simulink subsystem "CoolingControlRing_subsysref"  (R2020a)
settings: Solver=VariableStepAuto  StartTime=0.0  StopTime=10.0  RelTol=1e-3
libraries: inverter_loop_pump_and_fan_PWM_LVLibrary x1, motor_loop_pump_and_fan_PWM_LVLibrary x1, pump_and_fans_workingLibrary x1, inverter_loop_pump_and_fan_PWMLibrary x1, motor_loop_pump_and_fan_PWMLibrary x1, All_Sensors_Working x1
settings Model: Creator=Kiera  LastModifiedBy=Kiera

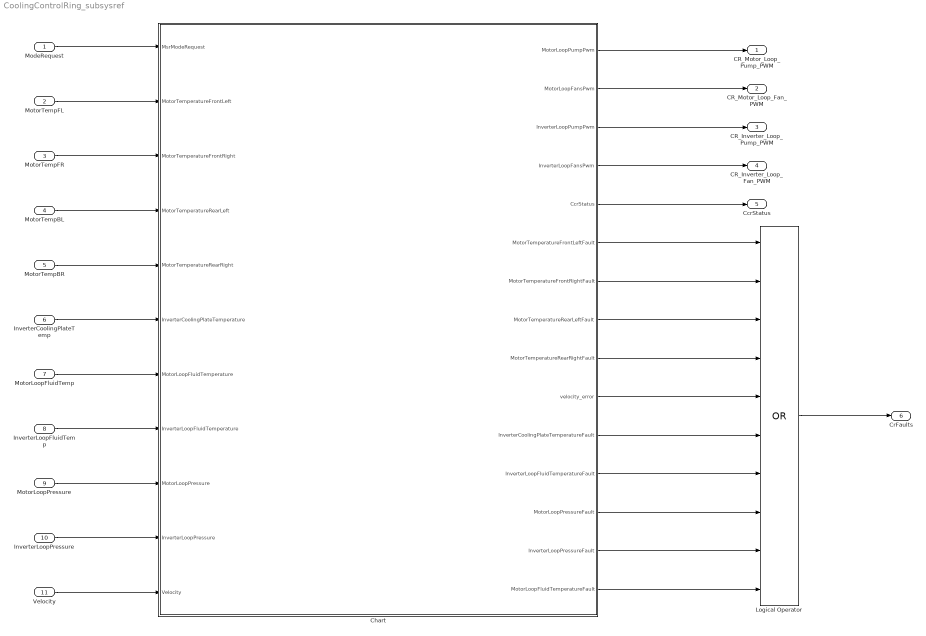
== system CoolingControlRing_subsysref ==
  ModeRequest : Inport
  MotorTempFL : Inport  Port=2
  MotorTempFR : Inport  Port=3
  MotorTempBL : Inport  Port=4
  MotorTempBR : Inport  Port=5
  InverterCoolingPlateTemp : Inport  Port=6
  MotorLoopFluidTemp : Inport  Port=7
  InverterLoopFluidTemp : Inport  Port=8
  MotorLoopPressure : Inport  Port=9
  InverterLoopPressure : Inport  Port=10
  Velocity : Inport  Port=11
  Chart : Stateflow chart  RequirementInfo={} %GIDa_8f277666_618f_4999_b577_53313bd8b4b0  TreatAsAtomicUnit=on
  Logical Operator : Logic  Operator=OR  Inputs=10  AllPortsSameDT=off  OutDataTypeStr=boolean
  CR_Motor_Loop_Pump_PWM : Outport  VectorParamsAs1DForOutWhenUnconnected=off
  CR_Motor_Loop_Fan_PWM : Outport  Port=2  VectorParamsAs1DForOutWhenUnconnected=off
  CR_Inverter_Loop_Pump_PWM : Outport  Port=3  VectorParamsAs1DForOutWhenUnconnected=off
  CR_Inverter_Loop_Fan_PWM : Outport  Port=4  VectorParamsAs1DForOutWhenUnconnected=off
  CcrStatus : Outport  Port=5  VectorParamsAs1DForOutWhenUnconnected=off
  CrFaults : Outport  Port=6  VectorParamsAs1DForOutWhenUnconnected=off
  wires:
  Chart/15(MotorLoopFluidTemperatureFault) -> Logical Operator/10
  Logical Operator/1 -> CrFaults/1
  MotorLoopFluidTemp/1 -> Chart/7(MotorLoopFluidTemperature)
  Chart/10(velocity_error) -> Logical Operator/5
  Chart/11(InverterCoolingPlateTemperatureFault) -> Logical Operator/6
  Chart/13(MotorLoopPressureFault) -> Logical Operator/8
  InverterCoolingPlateTemp/1 -> Chart/6(InverterCoolingPlateTemperature)
  Chart/12(InverterLoopFluidTemperatureFault) -> Logical Operator/7
  Chart/6(MotorTemperatureFrontLeftFault) -> Logical Operator/1
  ModeRequest/1 -> Chart/1(MsrModeRequest)
  MotorTempBL/1 -> Chart/4(MotorTemperatureRearLeft)
  Chart/3(InverterLoopPumpPwm) -> CR_Inverter_Loop_Pump_PWM/1
  Chart/2(MotorLoopFansPwm) -> CR_Motor_Loop_Fan_PWM/1
  InverterLoopPressure/1 -> Chart/10(InverterLoopPressure)
  MotorTempBR/1 -> Chart/5(MotorTemperatureRearRight)
  Chart/8(MotorTemperatureRearLeftFault) -> Logical Operator/3
  MotorTempFL/1 -> Chart/2(MotorTemperatureFrontLeft)
  Chart/1(MotorLoopPumpPwm) -> CR_Motor_Loop_Pump_PWM/1
  Chart/14(InverterLoopPressureFault) -> Logical Operator/9
  Chart/4(InverterLoopFansPwm) -> CR_Inverter_Loop_Fan_PWM/1
  Chart/5(CcrStatus) -> CcrStatus/1
  Chart/9(MotorTemperatureRearRightFault) -> Logical Operator/4
  InverterLoopFluidTemp/1 -> Chart/8(InverterLoopFluidTemperature)
  MotorTempFR/1 -> Chart/3(MotorTemperatureFrontRight)
  Chart/7(MotorTemperatureFrontRightFault) -> Logical Operator/2
  MotorLoopPressure/1 -> Chart/9(MotorLoopPressure)
  Velocity/1 -> Chart/11(Velocity)

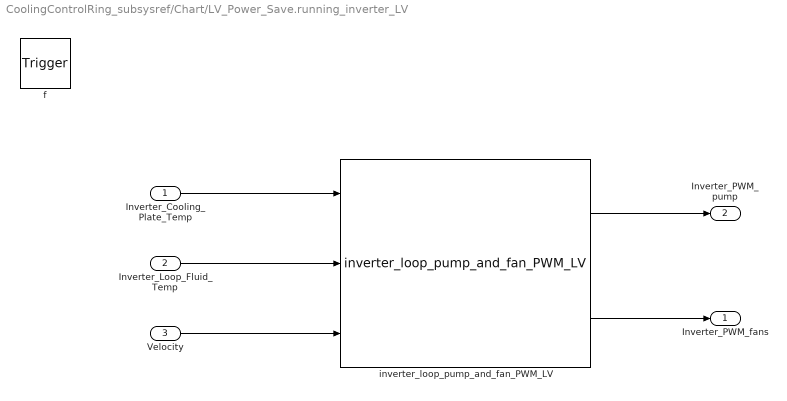
== system CoolingControlRing_subsysref/Chart/LV_Power_Save.running_inverter_LV ==
  Inverter_Cooling_Plate_Temp : Inport  OutDataTypeStr=double  PortDimensions=1
  Inverter_Loop_Fluid_Temp : Inport  Port=2  OutDataTypeStr=double  PortDimensions=1
  Velocity : Inport  Port=3  OutDataTypeStr=double  PortDimensions=1
  f : TriggerPort  TriggerType=function-call  VariantControl=Variant
      settings: CopyFcn=Stateflow.SLINSF.SimulinkMan.removeBlockPreDeleteFcn  PreDeleteFcn=Stateflow.SLINSF.SimulinkMan.unsafePredeleteFcn
  inverter_loop_pump_and_fan_PWM_LV : inverter_loop_pump_and_fan_PWM_LVLibrary/inverter_loop_pump_and_fan_PWM_LV  SystemSampleTime=-1  Latency=0  AutoFrameSizeCalculation=off
  Inverter_PWM_fans : Outport  VectorParamsAs1DForOutWhenUnconnected=off
  Inverter_PWM_pump : Outport  Port=2  VectorParamsAs1DForOutWhenUnconnected=off
  wires:
  inverter_loop_pump_and_fan_PWM_LV/2 -> Inverter_PWM_fans/1
  inverter_loop_pump_and_fan_PWM_LV/1 -> Inverter_PWM_pump/1
  Velocity/1 -> inverter_loop_pump_and_fan_PWM_LV/3
  Inverter_Cooling_Plate_Temp/1 -> inverter_loop_pump_and_fan_PWM_LV/1
  Inverter_Loop_Fluid_Temp/1 -> inverter_loop_pump_and_fan_PWM_LV/2

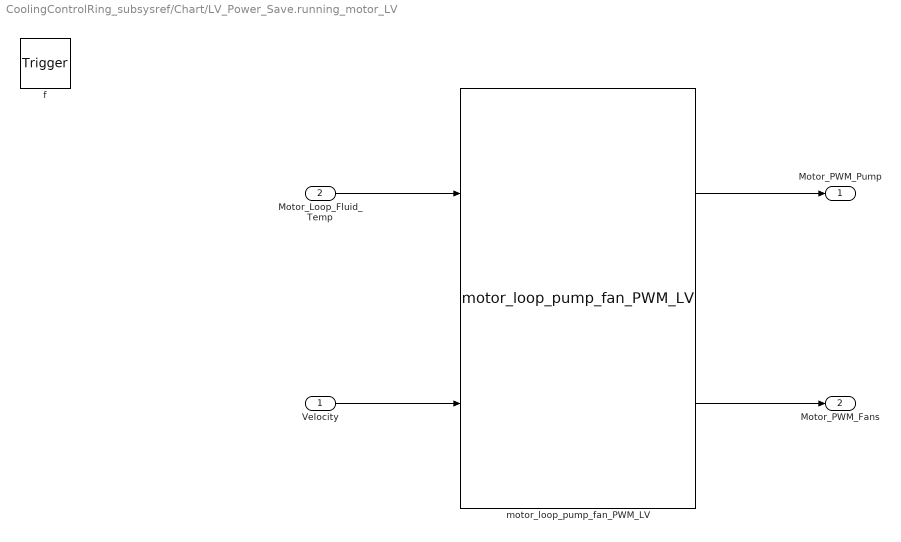
== system CoolingControlRing_subsysref/Chart/LV_Power_Save.running_motor_LV ==
  Velocity : Inport  OutDataTypeStr=double  PortDimensions=1
  Motor_Loop_Fluid_Temp : Inport  Port=2  OutDataTypeStr=double  PortDimensions=1
  f : TriggerPort  TriggerType=function-call  VariantControl=Variant
      settings: CopyFcn=Stateflow.SLINSF.SimulinkMan.removeBlockPreDeleteFcn  PreDeleteFcn=Stateflow.SLINSF.SimulinkMan.unsafePredeleteFcn
  motor_loop_pump_fan_PWM_LV : motor_loop_pump_and_fan_PWM_LVLibrary/motor_loop_pump_fan_PWM_LV  SystemSampleTime=-1  Latency=0  AutoFrameSizeCalculation=off
  Motor_PWM_Pump : Outport  OutDataTypeStr=double  PortDimensions=1  VectorParamsAs1DForOutWhenUnconnected=off
  Motor_PWM_Fans : Outport  Port=2  OutDataTypeStr=double  PortDimensions=1  VectorParamsAs1DForOutWhenUnconnected=off
  wires:
  Velocity/1 -> motor_loop_pump_fan_PWM_LV/2
  Motor_Loop_Fluid_Temp/1 -> motor_loop_pump_fan_PWM_LV/1
  motor_loop_pump_fan_PWM_LV/2 -> Motor_PWM_Fans/1
  motor_loop_pump_fan_PWM_LV/1 -> Motor_PWM_Pump/1

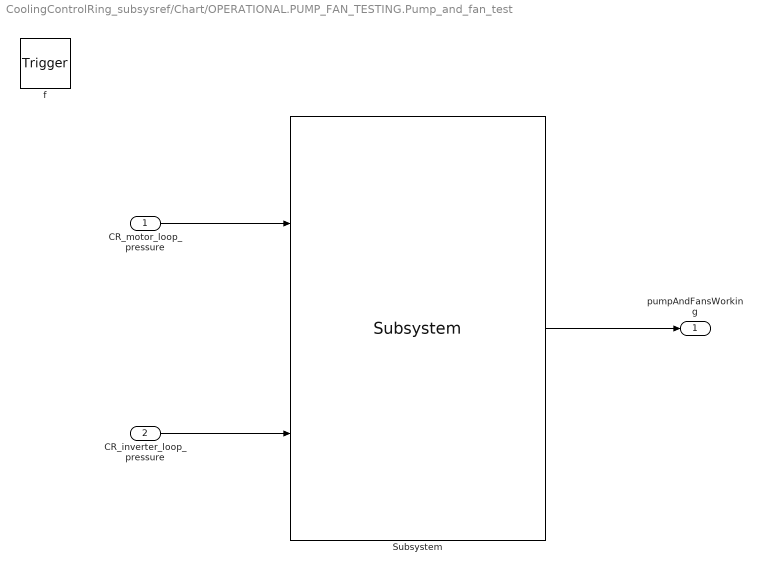
== system CoolingControlRing_subsysref/Chart/OPERATIONAL.PUMP_FAN_TESTING.Pump_and_fan_test ==
  CR_motor_loop_pressure : Inport  OutDataTypeStr=double  PortDimensions=1
  CR_inverter_loop_pressure : Inport  Port=2  OutDataTypeStr=double  PortDimensions=1
  f : TriggerPort  TriggerType=function-call  VariantControl=Variant
      settings: CopyFcn=Stateflow.SLINSF.SimulinkMan.removeBlockPreDeleteFcn  PreDeleteFcn=Stateflow.SLINSF.SimulinkMan.unsafePredeleteFcn
  Subsystem : pump_and_fans_workingLibrary/Subsystem  SystemSampleTime=-1  Latency=0  AutoFrameSizeCalculation=off
  pumpAndFansWorking : Outport  VectorParamsAs1DForOutWhenUnconnected=off
  wires:
  Subsystem/1 -> pumpAndFansWorking/1
  CR_inverter_loop_pressure/1 -> Subsystem/2
  CR_motor_loop_pressure/1 -> Subsystem/1

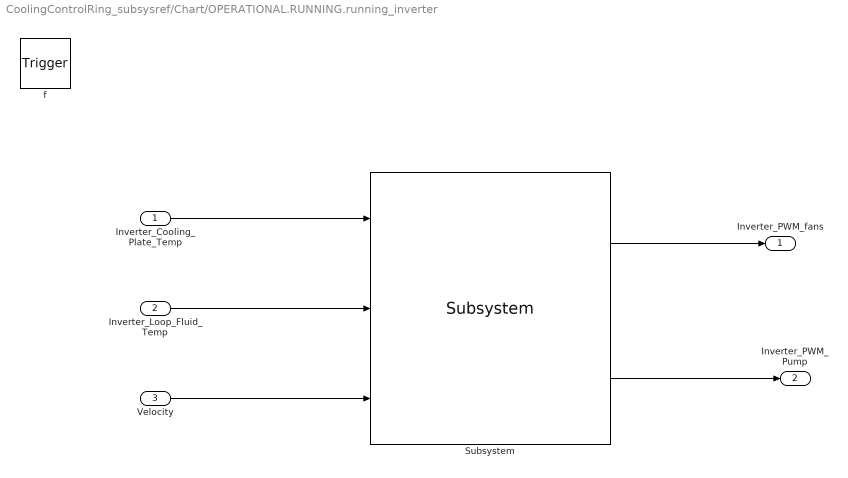
== system CoolingControlRing_subsysref/Chart/OPERATIONAL.RUNNING.running_inverter ==
  Inverter_Cooling_Plate_Temp : Inport  OutDataTypeStr=double  PortDimensions=1
  Inverter_Loop_Fluid_Temp : Inport  Port=2  OutDataTypeStr=double  PortDimensions=1
  Velocity : Inport  Port=3  OutDataTypeStr=double  PortDimensions=1
  f : TriggerPort  TriggerType=function-call  VariantControl=Variant
      settings: CopyFcn=Stateflow.SLINSF.SimulinkMan.removeBlockPreDeleteFcn  PreDeleteFcn=Stateflow.SLINSF.SimulinkMan.unsafePredeleteFcn
  Subsystem : inverter_loop_pump_and_fan_PWMLibrary/Subsystem  SystemSampleTime=-1  Latency=0  AutoFrameSizeCalculation=off
  Inverter_PWM_fans : Outport  OutDataTypeStr=double  PortDimensions=1  VectorParamsAs1DForOutWhenUnconnected=off
  Inverter_PWM_Pump : Outport  Port=2  OutDataTypeStr=double  PortDimensions=1  VectorParamsAs1DForOutWhenUnconnected=off
  wires:
  Subsystem/1 -> Inverter_PWM_fans/1
  Subsystem/2 -> Inverter_PWM_Pump/1
  Velocity/1 -> Subsystem/3
  Inverter_Loop_Fluid_Temp/1 -> Subsystem/2
  Inverter_Cooling_Plate_Temp/1 -> Subsystem/1

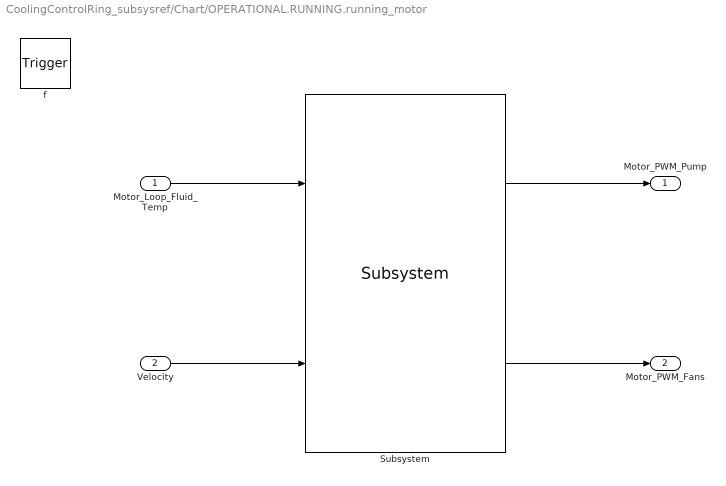
== system CoolingControlRing_subsysref/Chart/OPERATIONAL.RUNNING.running_motor ==
  Motor_Loop_Fluid_Temp : Inport  OutDataTypeStr=double  PortDimensions=1
  Velocity : Inport  Port=2  OutDataTypeStr=double  PortDimensions=1
  f : TriggerPort  TriggerType=function-call  VariantControl=Variant
      settings: CopyFcn=Stateflow.SLINSF.SimulinkMan.removeBlockPreDeleteFcn  PreDeleteFcn=Stateflow.SLINSF.SimulinkMan.unsafePredeleteFcn
  Subsystem : motor_loop_pump_and_fan_PWMLibrary/Subsystem  SystemSampleTime=-1  Latency=0  AutoFrameSizeCalculation=off
  Motor_PWM_Pump : Outport  OutDataTypeStr=double  PortDimensions=1  VectorParamsAs1DForOutWhenUnconnected=off
  Motor_PWM_Fans : Outport  Port=2  OutDataTypeStr=double  PortDimensions=1  VectorParamsAs1DForOutWhenUnconnected=off
  wires:
  Motor_Loop_Fluid_Temp/1 -> Subsystem/1
  Velocity/1 -> Subsystem/2
  Subsystem/2 -> Motor_PWM_Fans/1
  Subsystem/1 -> Motor_PWM_Pump/1

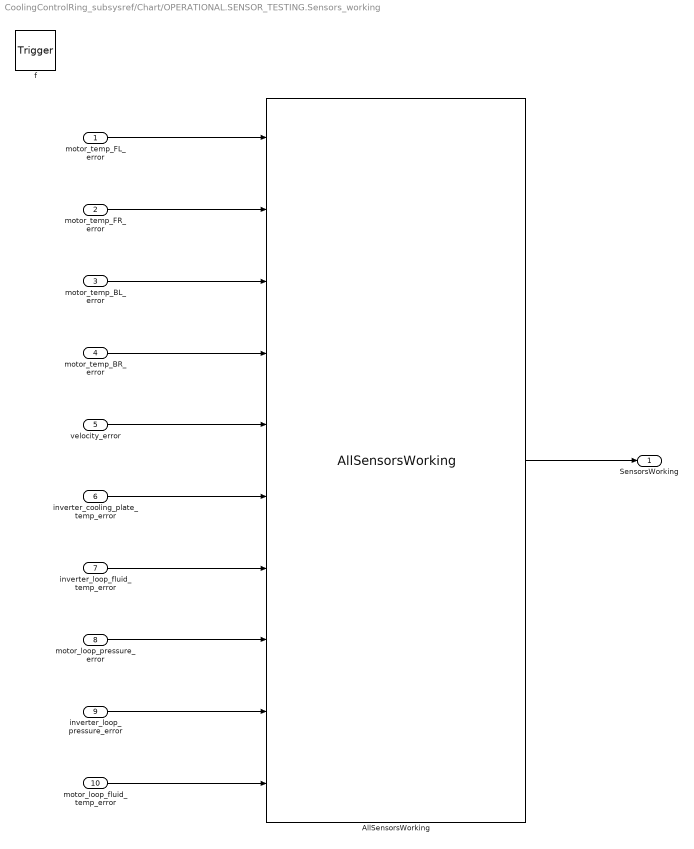
== system CoolingControlRing_subsysref/Chart/OPERATIONAL.SENSOR_TESTING.Sensors_working ==
  motor_temp_FL_error : Inport  OutDataTypeStr=double  PortDimensions=1
  motor_temp_FR_error : Inport  Port=2  OutDataTypeStr=double  PortDimensions=1
  motor_temp_BL_error : Inport  Port=3  OutDataTypeStr=double  PortDimensions=1
  motor_temp_BR_error : Inport  Port=4  OutDataTypeStr=double  PortDimensions=1
  velocity_error : Inport  Port=5  OutDataTypeStr=double  PortDimensions=1
  inverter_cooling_plate_temp_error : Inport  Port=6  OutDataTypeStr=double  PortDimensions=1
  inverter_loop_fluid_temp_error : Inport  Port=7  OutDataTypeStr=double  PortDimensions=1
  motor_loop_pressure_error : Inport  Port=8  OutDataTypeStr=double  PortDimensions=1
  inverter_loop_pressure_error : Inport  Port=9  OutDataTypeStr=double  PortDimensions=1
  motor_loop_fluid_temp_error : Inport  Port=10  OutDataTypeStr=double  PortDimensions=1
  f : TriggerPort  TriggerType=function-call  VariantControl=Variant
      settings: CopyFcn=Stateflow.SLINSF.SimulinkMan.removeBlockPreDeleteFcn  PreDeleteFcn=Stateflow.SLINSF.SimulinkMan.unsafePredeleteFcn
  AllSensorsWorking : All_Sensors_Working/AllSensorsWorking  SystemSampleTime=-1  Latency=0  AutoFrameSizeCalculation=off
  SensorsWorking : Outport  VectorParamsAs1DForOutWhenUnconnected=off
  wires:
  motor_loop_fluid_temp_error/1 -> AllSensorsWorking/10
  inverter_loop_pressure_error/1 -> AllSensorsWorking/9
  motor_loop_pressure_error/1 -> AllSensorsWorking/8
  inverter_loop_fluid_temp_error/1 -> AllSensorsWorking/7
  inverter_cooling_plate_temp_error/1 -> AllSensorsWorking/6
  velocity_error/1 -> AllSensorsWorking/5
  motor_temp_BR_error/1 -> AllSensorsWorking/4
  motor_temp_BL_error/1 -> AllSensorsWorking/3
  motor_temp_FL_error/1 -> AllSensorsWorking/1
  motor_temp_FR_error/1 -> AllSensorsWorking/2
  AllSensorsWorking/1 -> SensorsWorking/1

== stateflow chart CoolingControlRing_subsysref/Chart ==
  state OFF
    entry:
    MotorLoopPumpPwm=0;
    MotorLoopFansPwm=0;
    InverterLoopPumpPwm=0;
    InverterLoopFansPwm=0;
    CcrStatus = RING_STATUS.OFF;
    SensorSanity;
  state SHUTDOWN
    entry:
    CcrStatus = RING_STATUS.SHUTDOWN_COMPLETE_LV;
    % shutdown cooling fans and pump
  state OPERATIONAL
    entry:
    CcrStatus = RING_STATUS.SHUTDOWN_IN_PROGRESS_LV;
    state RUNNING
      entry:
      CcrStatus = RING_STATUS.RUNNING;
      during:
      [MotorLoopPumpPwm,MotorLoopFansPwm] = running_motor(MotorLoopFluidTemperature,Velocity)
      [InverterLoopFansPwm,InverterLoopPumpPwm] = running_inverter(InverterCoolingPlateTemperature,InverterLoopFluidTemperature,Velocity)
      state [Motor_PWM_Pump,Motor_PWM_Fans] = running_motor(Motor_Loop_Fluid_Temp,Velocity) [function]
      state [Inverter_PWM_fans,Inverter_PWM_Pump] = running_inverter(Inverter_Cooling_Plate_Temp,Inverter_Loop_Fluid_Temp,Velocity) [function]
    state TestingComplete
      entry:
      CcrStatus = RING_STATUS.STARTUP_COMPLETE_LV;
    state SENSOR_TESTING
      % sanity test on signal inputs
      % ensure sensor output values are within reasonable range
      entry:
      sensorsWorking=0;
      during:
      SensorSanity;
      sensorsWorking = Sensors_working(MotorTemperatureFrontLeftFault,MotorTemperatureFrontRightFault,MotorTemperatureRearLeftFault,MotorTemperatureRearRightFault,velocity_error,InverterCoolingPlateTemperatureFault,MotorLoopFluidTemperatureFault,InverterLoopFluidTemperatureFault,MotorLoopPressureFault,InverterLoopPressureFault);
      state SensorsWorking = Sensors_working(motor_temp_FL_error,motor_temp_FR_error,motor_temp_BL_error,motor_temp_BR_error,velocity_error,inverter_cooling_plate_temp_error,inverter_loop_fluid_temp_error,motor_loop_pressure_error,inverter_loop_pressure_error,motor_loop_fluid_temp_error) [function]
    state PUMP_FAN_TESTING
      % turning pump on and ensuring pressure ~=0
      % turning fans on and ensuring RPM ~=0
      entry:
      pumpAndFansWorking = 0;
      MotorLoopPumpPwm = CR.Motor_Testing_PWM_Pump;
      MotorLoopFansPwm = CR.Motor_Testing_PWM_Fans;
      InverterLoopPumpPwm = CR.Inverter_Testing_PWM_Pump;
      InverterLoopFansPwm = CR.Inverter_Testing_PWM_Fans;
      during:
      pumpAndFansWorking = Pump_and_fan_test(MotorLoopPressure,InverterLoopPressure)
      state pumpAndFansWorking = Pump_and_fan_test(CR_motor_loop_pressure,CR_inverter_loop_pressure) [function]
    (default) -> SENSOR_TESTING
    TestingComplete -> RUNNING : [MsrModeRequest == MSR_REQUEST.RUNNING]
    SENSOR_TESTING -> PUMP_FAN_TESTING : [sensorsWorking == 1]
    PUMP_FAN_TESTING -> TestingComplete : [pumpAndFansWorking == 1]
  state LV_Power_Save [commented out]
    entry:
    CcrStatus = CR.State.Running_LV;
    during:
    [MotorLoopPumpPwm,MotorLoopFansPwm] = running_motor_LV(Velocity,MotorLoopFluidTemperature)
    [InverterLoopFansPwm,InverterLoopPumpPwm] = running_inverter_LV(InverterCoolingPlateTemperature,InverterLoopFluidTemperature,Velocity)
    state [Motor_PWM_Pump,Motor_PWM_Fans] = running_motor_LV(Velocity,Motor_Loop_Fluid_Temp) [function] [commented out]
    state [Inverter_PWM_fans,Inverter_PWM_pump] = running_inverter_LV(Inverter_Cooling_Plate_Temp,Inverter_Loop_Fluid_Temp,Velocity) [function] [commented out]
  (default) -> OFF
  SHUTDOWN -> OFF : [MsrModeRequest == MSR_REQUEST.OFF]
  OPERATIONAL -> SHUTDOWN : [MsrModeRequest == MSR_REQUEST.SHUTDOWN_LV]
  OFF -> OPERATIONAL : [MsrModeRequest == MSR_REQUEST.STARTUP_LV]
  data: Motor_Loop_Fluid_Temp function_input double size=1; Velocity function_input double size=1; Motor_PWM_Pump function_output double size=1; Motor_PWM_Fans function_output double size=1; Inverter_Cooling_Plate_Temp function_input double size=1; Inverter_Loop_Fluid_Temp function_input double size=1; Velocity function_input double size=1; Inverter_PWM_fans function_output double size=1; Inverter_PWM_Pump function_output double size=1; SensorsWorking function_output; motor_temp_FL_error function_input double size=1; motor_temp_FR_error function_input double size=1; motor_temp_BL_error function_input double size=1; motor_temp_BR_error function_input double size=1; velocity_error function_input double size=1; inverter_cooling_plate_temp_error function_input double size=1; inverter_loop_fluid_temp_error function_input double size=1; motor_loop_pressure_error function_input double size=1; inverter_loop_pressure_error function_input double size=1; motor_loop_fluid_temp_error function_input double size=1; CR_motor_loop_pressure function_input double size=1; CR_inverter_loop_pressure function_input double size=1; pumpAndFansWorking function_output; Velocity function_input double size=1; Motor_PWM_Pump function_output double size=1; Motor_PWM_Fans function_output double size=1; Motor_Loop_Fluid_Temp function_input double size=1; Inverter_Cooling_Plate_Temp function_input double size=1; Inverter_Loop_Fluid_Temp function_input double size=1; Velocity function_input double size=1; Inverter_PWM_fans function_output double size=1; Inverter_PWM_pump function_output double size=1; MsrModeRequest input Enum: MSR_REQUEST; MotorLoopPumpPwm output double; MotorLoopFansPwm output double; InverterLoopPumpPwm output; InverterLoopFansPwm output; MotorTemperatureFrontLeft input; MotorTemperatureFrontRight input; MotorTemperatureRearLeft input; MotorTemperatureRearRight input; InverterCoolingPlateTemperature input; MotorLoopFluidTemperature input; InverterLoopFluidTemperature input; MotorLoopPressure input; InverterLoopPressure input; Velocity input; CcrStatus output Enum: RING_STATUS; CR parameter; MotorTemperatureFrontLeftFault output; MotorTemperatureFrontRightFault output; MotorTemperatureRearLeftFault output; MotorTemperatureRearRightFault output; velocity_error output; InverterCoolingPlateTemperatureFault output; InverterLoopFluidTemperatureFault output; MotorLoopPressureFault output; InverterLoopPressureFault output; sensorsWorking local; pumpAndFansWorking local; MotorLoopFluidTemperatureFault output
  function SensorSanity:
    | function SensorSanity
    | if (MotorTemperatureFrontLeft > CR.motor_temp_max || MotorTemperatureFrontLeft < CR.motor_temp_min)
    |     MotorTemperatureFrontLeftFault = CR.ERROR.FAILURE;
    | else
    |     MotorTemperatureFrontLeftFault = CR.ERROR.PASS;
    | end
    | 
    | if (MotorTemperatureFrontRight > CR.motor_temp_max || MotorTemperatureFrontRight < CR.motor_temp_min)
    |     MotorTemperatureFrontRightFault = CR.ERROR.FAILURE;
    | else
    |     MotorTemperatureFrontRightFault = CR.ERROR.PASS;
    | end
    | 
    | if (MotorTemperatureRearLeft > CR.motor_temp_max || MotorTemperatureRearLeft < CR.motor_temp_min)
    |     MotorTemperatureRearLeftFault = CR.ERROR.FAILURE;
    | else
    |     MotorTemperatureRearLeftFault = CR.ERROR.PASS;
    | end
    | 
    | if (MotorTemperatureRearRight > CR.motor_temp_max || MotorTemperatureRearRight < CR.motor_temp_min)
    |     MotorTemperatureRearRightFault = CR.ERROR.FAILURE;
    | else
    |     MotorTemperatureRearRightFault = CR.ERROR.PASS;
    | end
    | 
    | if (Velocity > CR.velocity_max || Velocity < CR.velocity_min)
    |     velocity_error = CR.ERROR.FAILURE;
    | else
    |     velocity_error = CR.ERROR.PASS;
    | end
    | 
    | if (InverterCoolingPlateTemperature > CR.inverter_cooling_plate_max || InverterCoolingPlateTemperature < CR.inverter_cooling_plate_min)
    |     InverterCoolingPlateTemperatureFault = CR.ERROR.FAILURE;
    | else
    |     InverterCoolingPlateTemperatureFault = CR.ERROR.PASS;
    | end
    | 
    | if (MotorLoopFluidTemperature > CR.motor_fluid_temp_max || MotorLoopFluidTemperature < CR.motor_fluid_temp_min)
    |     MotorLoopFluidTemperatureFault = CR.ERROR.FAILURE;
    | else
    |     MotorLoopFluidTemperatureFault = CR.ERROR.PASS;
    | end
    | 
    | if (InverterLoopFluidTemperature > CR.inverter_fluid_temp_max || InverterLoopFluidTemperature < CR.inverter_fluid_temp_min)
    |     InverterLoopFluidTemperatureFault = CR.ERROR.FAILURE;
    | else
    |     InverterLoopFluidTemperatureFault = CR.ERROR.PASS;
    | end
    | 
    | if (MotorLoopPressure > CR.motor_loop_pressure_max || MotorLoopPressure < CR.motor_loop_pressure_min)
    |     MotorLoopPressureFault = CR.ERROR.FAILURE;
    | else
    |     MotorLoopPressureFault = CR.ERROR.PASS;
    | end
    | 
    | if (InverterLoopPressure > CR.inverter_loop_pressure_max || InverterLoopPressure < CR.inverter_loop_pressure_min)
    |     InverterLoopPressureFault = CR.ERROR.FAILURE;
    | else
    |     InverterLoopPressureFault = CR.ERROR.PASS;
    | end
    | 
    | 
    | end
